simulink model "simu_control_robot_3"  (Simulink 7.9)
settings: Solver=ode3  StartTime=0  StopTime=1.2  FixedStep=1/100  RelTol=1e-3
values from neighbouring files (symbols this model uses):
  f = 200    [WPG_results.m]    (also in WPG_results_10.m = wpg_param.frequency; WPG_results_2.m = wpg_param.frequency; WPG_results_3.m = wpg_param.frequency; WPG_results_4.m = wpg_param.frequency)
  J1 = [J1;Jmat.step_1.J_tot((i-1)*6+1:(i-1)*6+6,:)]    [WPG_results_5.m]
  J1_inv = [J1_inv;J1(end-5:end,:)^-1]    [WPG_results_5.m]
  k1 = -q(1)*q(2)-1    [WPG_results.m]    (also in WPG_results_10.m; WPG_results_2.m; WPG_results_3.m; WPG_results_4.m)
  k2 = (q(1)+q(2))/-q(3)    [WPG_results.m]    (also in WPG_results_10.m; WPG_results_2.m; WPG_results_3.m; WPG_results_4.m)
  k3 = w    [WPG_results.m]    (also in WPG_results_10.m; WPG_results_2.m; WPG_results_3.m; WPG_results_4.m)
  traslx_1 = wpg_param.step_number_pankle_fixed(1,2)-wpg_param.backtoankle    [WPG_results_10.m]    (also in WPG_results_2.m; WPG_results_3.m; WPG_results_4.m; WPG_results_5.m)
  trasly_1 = wpg_param.step_number_pankle_fixed(1,3)-(Lfooty/2-wpg_param.inttoankle)    [WPG_results_10.m]    (also in WPG_results_2.m; WPG_results_3.m; WPG_results_4.m; WPG_results_5.m)
  w = wpg_param.w    [WPG_results.m]    (also in WPG_results_10.m; WPG_results_2.m; WPG_results_3.m; WPG_results_4.m)
  xsx_d = repmat(0,duration_disc,1)    [WPG_results_10.m]    (also in WPG_results_2.m = zmp.A_xcom_spd(1:sum(wpg_param.discretization(1:wpg_param.nb; WPG_results_3.m = zmp.A_xcom_spd(1:sum(wpg_param.discretization(1:wpg_param.nb; WPG_results_4.m = repmat(zmp.A_xcom_spd(1,:)*wpg_param.psa_abcdDSP(1:size(zmp.; WPG_results_5.m = [time xsx_d-xsx_d_init])
  xx_d = repmat(trajectories_zmp.xpcom(1),duration_disc,1)    [WPG_results_10.m]    (also in WPG_results_2.m = trajectories_zmp.xpcom(1:sum(wpg_param.discretization(1:wpg_; WPG_results_3.m = trajectories_zmp.xpcom(1:sum(wpg_param.discretization(1:wpg_; WPG_results_4.m; WPG_results_5.m = [time xx_d-xx_d_init])
  ysx_d = repmat(0,duration_disc,1)    [WPG_results_10.m]    (also in WPG_results_2.m = zmp.A_ycom_spd(1:sum(wpg_param.discretization(1:wpg_param.nb; WPG_results_3.m = zmp.A_ycom_spd(1:sum(wpg_param.discretization(1:wpg_param.nb; WPG_results_4.m = repmat(zmp.A_ycom_spd(1,:)*wpg_param.psa_abcdDSP(end/2+1:end; WPG_results_5.m = [time ysx_d-ysx_d_init])
  yx_d = repmat(0,duration_disc,1)    [WPG_results_10.m]    (also in WPG_results_2.m = trajectories_zmp.ypcom(1:sum(wpg_param.discretization(1:wpg_; WPG_results_3.m = trajectories_zmp.ypcom(1:sum(wpg_param.discretization(1:wpg_; WPG_results_4.m = repmat(trajectories_zmp.ypcom(1),duration_disc,1); WPG_results_5.m = [time yx_d-yx_d_init])
undefined symbols (not defined in the file or in its folder): Jmat, wpg_param
settings Model: Creator=pajon  LastModifiedBy=pajon

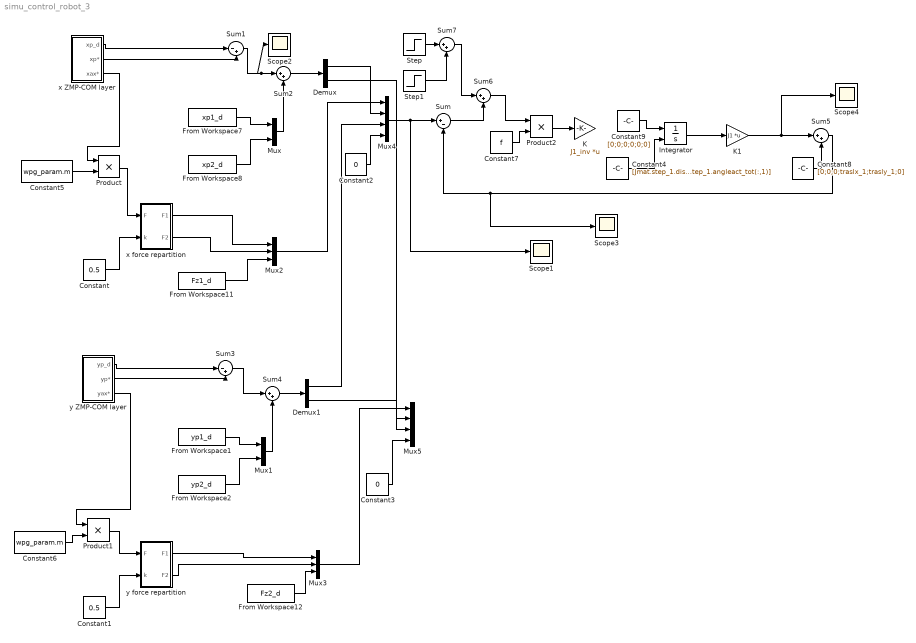
== system simu_control_robot_3 ==
  Constant : Constant  Value=0.5
  Constant1 : Constant  Value=0.5
  Constant2 : Constant  Value=0
  Constant3 : Constant  Value=0
  Constant4 : Constant  Value=[Jmat.step_1.displ_tot(:,1);Jmat.step_1.angleact_tot(:,1)]  VectorParams1D=off
  Constant5 : Constant  Value=wpg_param.m
  Constant6 : Constant  Value=wpg_param.m
  Constant7 : Constant  Value=f
  Constant8 : Constant  Value=[0;0;0;traslx_1;trasly_1;0]
  Constant9 : Constant  Value=[0;0;0;0;0;0]
  Demux : Demux  Outputs=2
  Demux1 : Demux  Outputs=2
  From Workspace1 : FromWorkspace  VariableName=yp1_d  SampleTime=0
  From Workspace11 : FromWorkspace  VariableName=Fz1_d  SampleTime=0
  From Workspace12 : FromWorkspace  VariableName=Fz2_d  SampleTime=0
  From Workspace2 : FromWorkspace  VariableName=yp2_d  SampleTime=0
  From Workspace7 : FromWorkspace  VariableName=xp1_d  SampleTime=0
  From Workspace8 : FromWorkspace  VariableName=xp2_d  SampleTime=0
  Integrator : Integrator  InitialConditionSource=external
  K : Gain  Gain=J1_inv  Multiplication=Matrix(K*u)
  K1 : Gain  Gain=J1  Multiplication=Matrix(K*u)
  Mux : Mux  Inputs=2
  Mux1 : Mux  Inputs=2
  Mux2 : Mux  Inputs=3
  Mux3 : Mux  Inputs=3
  Mux4 : Mux
  Mux5 : Mux
  Product : Product  RndMeth=Zero
  Product1 : Product  RndMeth=Zero
  Product2 : Product  RndMeth=Zero
  Scope{1..4} (4 alike) : Scope
      Scope1 settings: SaveName=ScopeData2
      Scope3 settings: SaveName=ScopeData3
      Scope4 settings: SaveName=ScopeData4
  Step : Step  Time=0.4  Before=[0;0;0;0;0;0]  After=[5;0;0;0.02;0;0]  SampleTime=0
  Step1 : Step  Time=0.8  Before=[0;0;0;0;0;0]  After=[5;0;0;0.02;0;0]*(-1)  SampleTime=0
  Sum : Sum  Inputs=|+-
  Sum1 : Sum  Inputs=|-+
  Sum{2,4..7} (5 alike) : Sum  Inputs=|++
  Sum3 : Sum  Inputs=|-+
  x ZMP-COM layer : Subsystem
  x force repartition : Subsystem
  y ZMP-COM layer : Subsystem
  y force repartition : Subsystem
  wires:
  From Workspace7/1 -> Mux/1
  From Workspace8/1 -> Mux/2
  Mux/1 -> Sum2/2
  x ZMP-COM layer/1(xp_d) -> Sum1/1
  x ZMP-COM layer/2(xp*) -> Sum1/2
  Sum1/1 -> Sum2/1, Scope2/1
  From Workspace1/1 -> Mux1/1
  From Workspace2/1 -> Mux1/2
  Mux1/1 -> Sum4/2
  Sum3/1 -> Sum4/1
  y ZMP-COM layer/1(yp_d) -> Sum3/1
  y ZMP-COM layer/2(yp*) -> Sum3/2
  Constant/1 -> x force repartition/2(k)
  Constant1/1 -> y force repartition/2(k)
  Sum4/1 -> Demux1/1
  Sum2/1 -> Demux/1
  Product/1 -> x force repartition/1(F)
  x ZMP-COM layer/3(xax*) -> Product/1
  Product1/1 -> y force repartition/1(F)
  y ZMP-COM layer/3(yax*) -> Product1/1
  Constant5/1 -> Product/2
  Constant6/1 -> Product1/2
  x force repartition/1(F1) -> Mux2/1
  x force repartition/2(F2) -> Mux2/2
  From Workspace11/1 -> Mux2/3
  y force repartition/1(F1) -> Mux3/1
  y force repartition/2(F2) -> Mux3/2
  From Workspace12/1 -> Mux3/3
  Mux2/1 -> Mux4/1
  Demux/1 -> Mux4/2
  Demux1/1 -> Mux4/3
  Mux3/1 -> Mux5/1
  Demux/2 -> Mux5/2
  Demux1/2 -> Mux5/3
  Constant2/1 -> Mux4/4
  Constant3/1 -> Mux5/4
  Constant4/1 -> Integrator/2
  Mux4/1 -> Sum/1, Scope1/1
  Constant7/1 -> Product2/2
  Product2/1 -> K/1
  Integrator/1 -> K1/1
  Constant8/1 -> Sum5/2
  Sum5/1 -> Sum/2, Scope3/1
  Sum6/1 -> Product2/1
  Sum/1 -> Sum6/2
  Step/1 -> Sum7/1
  Step1/1 -> Sum7/2
  Sum7/1 -> Sum6/1
  Constant9/1 -> Integrator/1
  K1/1 -> Sum5/1, Scope4/1

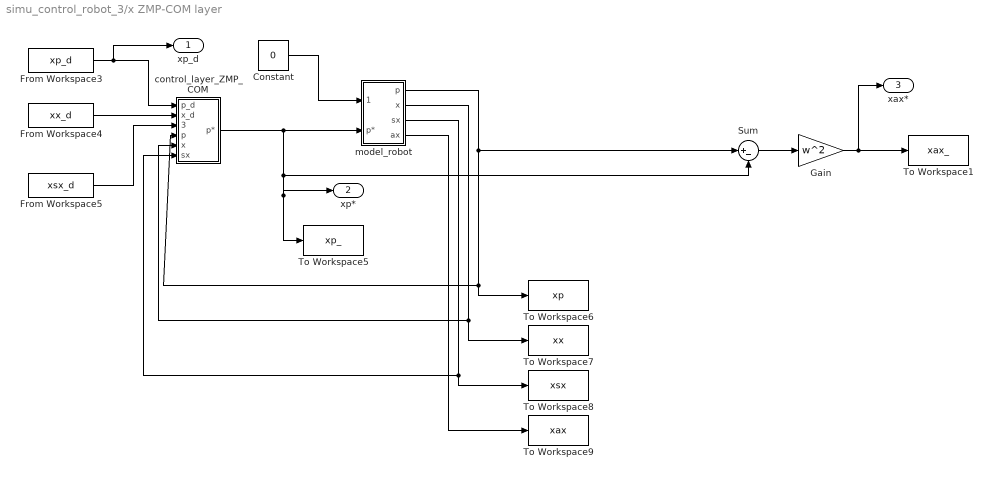
== system simu_control_robot_3/x ZMP-COM layer ==
  Constant : Constant  Value=0
  From Workspace3 : FromWorkspace  VariableName=xp_d  SampleTime=0
  From Workspace4 : FromWorkspace  VariableName=xx_d  SampleTime=0
  From Workspace5 : FromWorkspace  VariableName=xsx_d  SampleTime=0
  Gain : Gain  Gain=w^2
  Sum : Sum  Inputs=|+-
  To Workspace1 : ToWorkspace  VariableName=xax_  SampleTime=-1
  To Workspace5 : ToWorkspace  VariableName=xp_  SampleTime=-1
  To Workspace6 : ToWorkspace  VariableName=xp  SampleTime=-1
  To Workspace7 : ToWorkspace  VariableName=xx  SampleTime=-1
  To Workspace8 : ToWorkspace  VariableName=xsx  SampleTime=-1
  To Workspace9 : ToWorkspace  VariableName=xax  SampleTime=-1
  control_layer_ZMP_COM : Subsystem
  model_robot : Subsystem
  xp_d : Outport
  xp* : Outport  Port=2
  xax* : Outport  Port=3
  wires:
  Constant/1 -> model_robot/1(perturb)
  Gain/1 -> To Workspace1/1, xax*/1
  model_robot/4(ax) -> To Workspace9/1
  From Workspace5/1 -> control_layer_ZMP_COM/3(sx_d)
  From Workspace4/1 -> control_layer_ZMP_COM/2(x_d)
  From Workspace3/1 -> control_layer_ZMP_COM/1(p_d), xp_d/1
  control_layer_ZMP_COM/1(p*) -> model_robot/2(p*), Sum/2, To Workspace5/1, xp*/1
  model_robot/1(p) -> control_layer_ZMP_COM/4(p), To Workspace6/1, Sum/1
  model_robot/2(x) -> control_layer_ZMP_COM/5(x), To Workspace7/1
  model_robot/3(sx) -> control_layer_ZMP_COM/6(sx), To Workspace8/1
  Sum/1 -> Gain/1

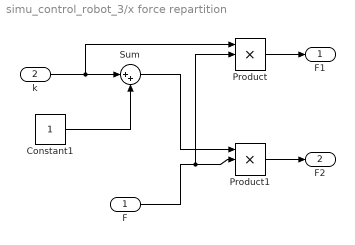
== system simu_control_robot_3/x force repartition ==
  F : Inport
  k : Inport  Port=2
  Constant1 : Constant
  Product : Product  Inputs=3  RndMeth=Zero
  Product1 : Product  Inputs=3  RndMeth=Zero
  Sum : Sum  Inputs=|++
  F1 : Outport
  F2 : Outport  Port=2
  wires:
  k/1 -> Sum/1, Product/1
  Constant1/1 -> Sum/2
  Sum/1 -> Product1/1
  F/1 -> Product1/2, Product/2
  Product/1 -> F1/1
  Product1/1 -> F2/1

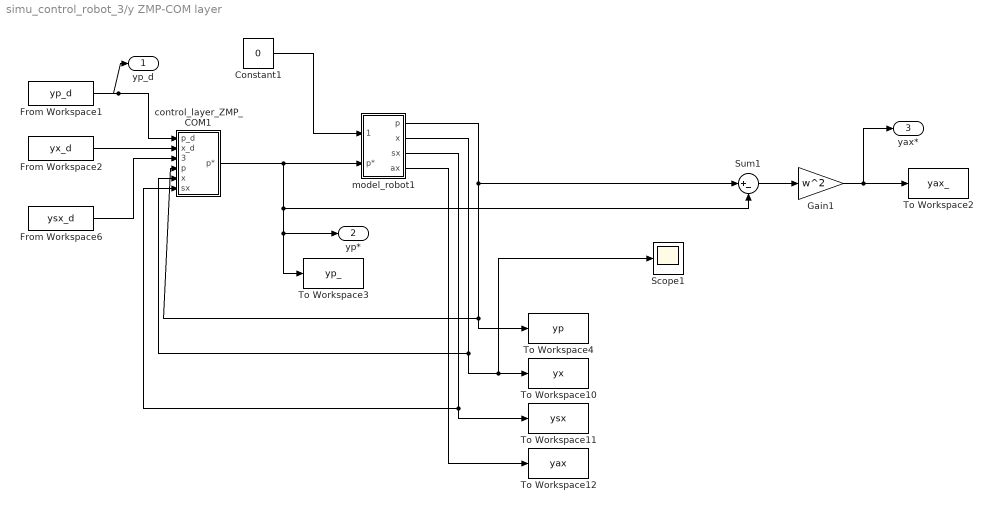
== system simu_control_robot_3/y ZMP-COM layer ==
  Constant1 : Constant  Value=0
  From Workspace1 : FromWorkspace  VariableName=yp_d  SampleTime=0
  From Workspace2 : FromWorkspace  VariableName=yx_d  SampleTime=0
  From Workspace6 : FromWorkspace  VariableName=ysx_d  SampleTime=0
  Gain1 : Gain  Gain=w^2
  Scope1 : Scope
  Sum1 : Sum  Inputs=|+-
  To Workspace10 : ToWorkspace  VariableName=yx  SampleTime=-1
  To Workspace11 : ToWorkspace  VariableName=ysx  SampleTime=-1
  To Workspace12 : ToWorkspace  VariableName=yax  SampleTime=-1
  To Workspace2 : ToWorkspace  VariableName=yax_  SampleTime=-1
  To Workspace3 : ToWorkspace  VariableName=yp_  SampleTime=-1
  To Workspace4 : ToWorkspace  VariableName=yp  SampleTime=-1
  control_layer_ZMP_COM1 : Subsystem
  model_robot1 : Subsystem
  yp_d : Outport
  yp* : Outport  Port=2
  yax* : Outport  Port=3
  wires:
  control_layer_ZMP_COM1/1(p*) -> model_robot1/2(p*), Sum1/2, To Workspace3/1, yp*/1
  From Workspace1/1 -> control_layer_ZMP_COM1/1(p_d), yp_d/1
  From Workspace2/1 -> control_layer_ZMP_COM1/2(x_d)
  From Workspace6/1 -> control_layer_ZMP_COM1/3(sx_d)
  model_robot1/1(p) -> To Workspace4/1, control_layer_ZMP_COM1/4(p), Sum1/1
  model_robot1/2(x) -> control_layer_ZMP_COM1/5(x), To Workspace10/1, Scope1/1
  model_robot1/3(sx) -> To Workspace11/1, control_layer_ZMP_COM1/6(sx)
  model_robot1/4(ax) -> To Workspace12/1
  Sum1/1 -> Gain1/1
  Gain1/1 -> To Workspace2/1, yax*/1
  Constant1/1 -> model_robot1/1(perturb)

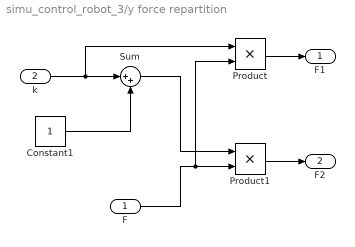
== system simu_control_robot_3/y force repartition ==
  F : Inport
  k : Inport  Port=2
  Constant1 : Constant
  Product : Product  RndMeth=Zero
  Product1 : Product  RndMeth=Zero
  Sum : Sum  Inputs=|++
  F1 : Outport
  F2 : Outport  Port=2
  wires:
  k/1 -> Sum/1, Product/1
  Constant1/1 -> Sum/2
  Sum/1 -> Product1/1
  F/1 -> Product1/2, Product/2
  Product/1 -> F1/1
  Product1/1 -> F2/1

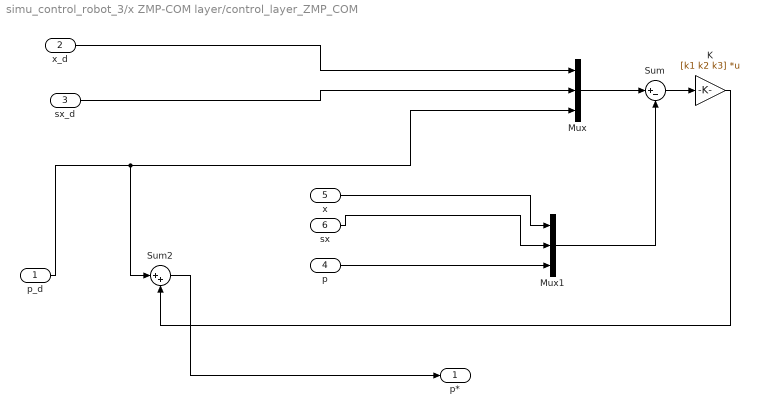
== system simu_control_robot_3/x ZMP-COM layer/control_layer_ZMP_COM ==
  p_d : Inport
  x_d : Inport  Port=2
  sx_d : Inport  Port=3
  p : Inport  Port=4
  x : Inport  Port=5
  sx : Inport  Port=6
  K : Gain  Gain=[k1 k2 k3]  Multiplication=Matrix(K*u)
  Mux : Mux  Inputs=3
  Mux1 : Mux  Inputs=3
  Sum : Sum  Inputs=|+-
  Sum2 : Sum  Inputs=|++
  p* : Outport
  wires:
  Mux/1 -> Sum/1
  Mux1/1 -> Sum/2
  Sum/1 -> K/1
  K/1 -> Sum2/2
  Sum2/1 -> p*/1
  x/1 -> Mux1/1
  sx/1 -> Mux1/2
  p_d/1 -> Mux/3, Sum2/1
  x_d/1 -> Mux/1
  sx_d/1 -> Mux/2
  p/1 -> Mux1/3

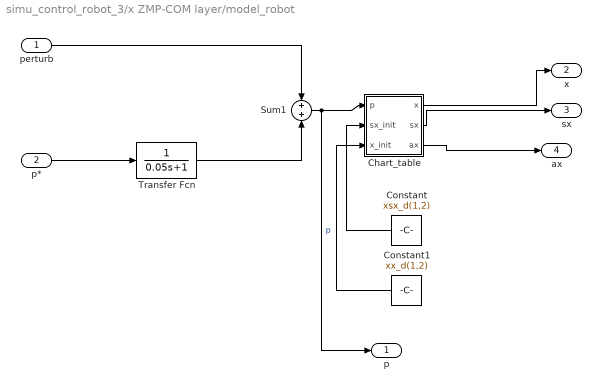
== system simu_control_robot_3/x ZMP-COM layer/model_robot ==
  perturb : Inport
  p* : Inport  Port=2
  Chart_table : Subsystem
  Constant : Constant  Value=xsx_d(1,2)
  Constant1 : Constant  Value=xx_d(1,2)
  Sum1 : Sum
  Transfer Fcn : TransferFcn  Denominator=[0.05 1]
  p : Outport
  x : Outport  Port=2
  sx : Outport  Port=3
  ax : Outport  Port=4
  wires:
  perturb/1 -> Sum1/1
  p*/1 -> Transfer Fcn/1
  Chart_table/1(x) -> x/1
  Chart_table/2(sx) -> sx/1
  Chart_table/3(ax) -> ax/1
  Transfer Fcn/1 -> Sum1/2
  Sum1/1 -> Chart_table/1(p), p/1  "p"
  Constant/1 -> Chart_table/2(sx_init)
  Constant1/1 -> Chart_table/3(x_init)

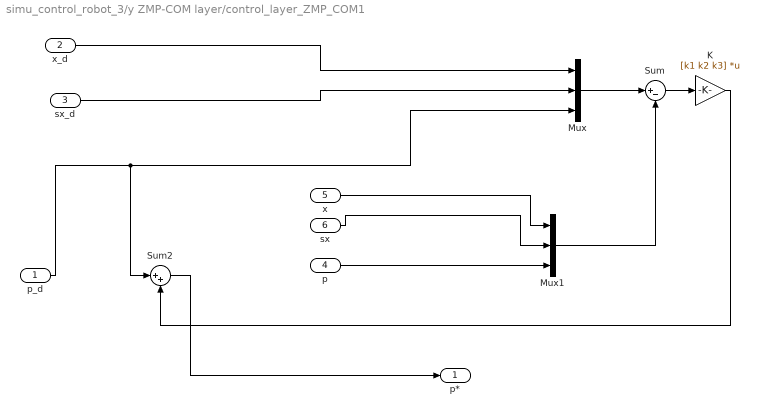
== system simu_control_robot_3/y ZMP-COM layer/control_layer_ZMP_COM1 ==
  p_d : Inport
  x_d : Inport  Port=2
  sx_d : Inport  Port=3
  p : Inport  Port=4
  x : Inport  Port=5
  sx : Inport  Port=6
  K : Gain  Gain=[k1 k2 k3]  Multiplication=Matrix(K*u)
  Mux : Mux  Inputs=3
  Mux1 : Mux  Inputs=3
  Sum : Sum  Inputs=|+-
  Sum2 : Sum  Inputs=|++
  p* : Outport
  wires:
  Mux/1 -> Sum/1
  Mux1/1 -> Sum/2
  Sum/1 -> K/1
  K/1 -> Sum2/2
  Sum2/1 -> p*/1
  x/1 -> Mux1/1
  sx/1 -> Mux1/2
  p_d/1 -> Mux/3, Sum2/1
  x_d/1 -> Mux/1
  sx_d/1 -> Mux/2
  p/1 -> Mux1/3

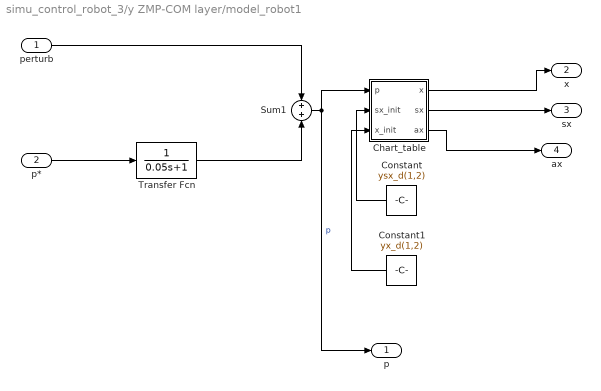
== system simu_control_robot_3/y ZMP-COM layer/model_robot1 ==
  perturb : Inport
  p* : Inport  Port=2
  Chart_table : Subsystem
  Constant : Constant  Value=ysx_d(1,2)
  Constant1 : Constant  Value=yx_d(1,2)
  Sum1 : Sum
  Transfer Fcn : TransferFcn  Denominator=[0.05 1]
  p : Outport
  x : Outport  Port=2
  sx : Outport  Port=3
  ax : Outport  Port=4
  wires:
  perturb/1 -> Sum1/1
  p*/1 -> Transfer Fcn/1
  Chart_table/1(x) -> x/1
  Chart_table/2(sx) -> sx/1
  Chart_table/3(ax) -> ax/1
  Transfer Fcn/1 -> Sum1/2
  Sum1/1 -> p/1, Chart_table/1(p)  "p"
  Constant/1 -> Chart_table/2(sx_init)
  Constant1/1 -> Chart_table/3(x_init)

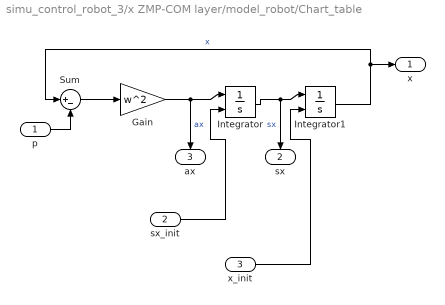
== system simu_control_robot_3/x ZMP-COM layer/model_robot/Chart_table ==
  p : Inport
  sx_init : Inport  Port=2
  x_init : Inport  Port=3
  Gain : Gain  Gain=w^2
  Integrator : Integrator  InitialConditionSource=external  InitialCondition=xsx_d(1,2)
  Integrator1 : Integrator  InitialConditionSource=external  InitialCondition=xx_d(1,2)
  Sum : Sum  Inputs=|+-
  x : Outport
  sx : Outport  Port=2
  ax : Outport  Port=3
  wires:
  Integrator/1 -> Integrator1/1, sx/1  "sx"
  Integrator1/1 -> Sum/1, x/1  "x"
  Gain/1 -> Integrator/1, ax/1  "ax"
  Sum/1 -> Gain/1
  p/1 -> Sum/2
  sx_init/1 -> Integrator/2
  x_init/1 -> Integrator1/2

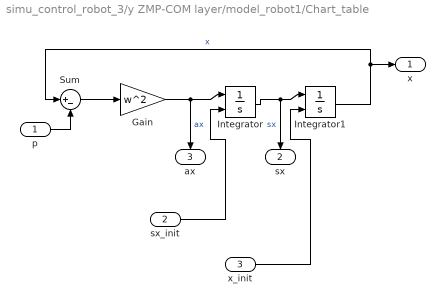
== system simu_control_robot_3/y ZMP-COM layer/model_robot1/Chart_table ==
  p : Inport
  sx_init : Inport  Port=2
  x_init : Inport  Port=3
  Gain : Gain  Gain=w^2
  Integrator : Integrator  InitialConditionSource=external  InitialCondition=xsx_d(1,2)
  Integrator1 : Integrator  InitialConditionSource=external  InitialCondition=xx_d(1,2)
  Sum : Sum  Inputs=|+-
  x : Outport
  sx : Outport  Port=2
  ax : Outport  Port=3
  wires:
  Integrator/1 -> Integrator1/1, sx/1  "sx"
  Integrator1/1 -> Sum/1, x/1  "x"
  Gain/1 -> Integrator/1, ax/1  "ax"
  Sum/1 -> Gain/1
  p/1 -> Sum/2
  sx_init/1 -> Integrator/2
  x_init/1 -> Integrator1/2
